simulink library "magnetometer_sim_lib"  (R2018b)
settings: Solver=VariableStepAuto  StartTime=0.0  StopTime=10.0  RelTol=1e-3
undefined symbols (not defined in the file): sim_params
libraries: simulink x3, dspmathops x2, aerolibutil x1
settings Model: Creator=colem  LastModifiedBy=colem

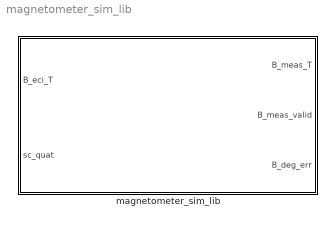
== system magnetometer_sim_lib ==
  magnetometer_sim_lib : Subsystem

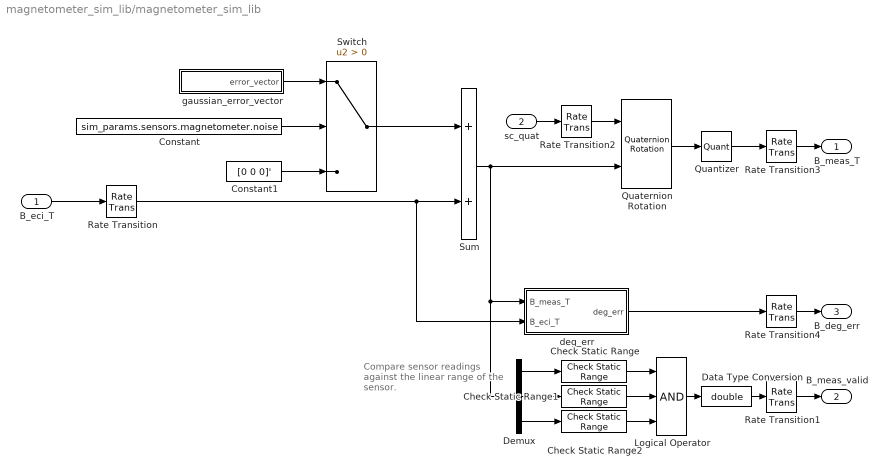
== system magnetometer_sim_lib/magnetometer_sim_lib ==
  note: Compare sensor readings
      | against the linear range
      | of the sensor.
  B_eci_T : Inport
  sc_quat : Inport  Port=2
  Check Static Range : simulink/Model Verification/Check  Static Range  Description=sim_params.sensors.magnetometer.B_min <= u <= sim_params.sensors.magnetometer.B_max  max=sim_params.sensors.magnetometer.B_max  max_included=on  min=sim_params.sensors.magnetometer.B_min  min_included=on  enabled=on  stopWhenAssertionFail=off  export=on  icon=text
      settings: SourceProductName=Simulink  SourceProductBaseCode=SL
  Check Static Range1 : simulink/Model Verification/Check  Static Range  Description=sim_params.sensors.magnetometer.B_min <= u <= sim_params.sensors.magnetometer.B_max  max=sim_params.sensors.magnetometer.B_max  max_included=on  min=sim_params.sensors.magnetometer.B_min  min_included=on  enabled=on  stopWhenAssertionFail=off  export=on  icon=graphic
      settings: SourceProductName=Simulink  SourceProductBaseCode=SL
  Check Static Range2 : simulink/Model Verification/Check  Static Range  Description=sim_params.sensors.magnetometer.B_min <= u <= sim_params.sensors.magnetometer.B_max  max=sim_params.sensors.magnetometer.B_max  max_included=on  min=sim_params.sensors.magnetometer.B_min  min_included=on  enabled=on  stopWhenAssertionFail=off  export=on  icon=graphic
      settings: SourceProductName=Simulink  SourceProductBaseCode=SL
  Constant : Constant  Value=sim_params.sensors.magnetometer.noise  SampleTime=sim_params.sensors.magnetometer.sample_time_s
  Constant1 : Constant  Value=[0 0 0]'  SampleTime=sim_params.sensors.magnetometer.sample_time_s
  Data Type Conversion : DataTypeConversion  OutDataTypeStr=double
  Demux : Demux  Outputs=3
  Logical Operator : Logic  Inputs=3  AllPortsSameDT=off  OutDataTypeStr=boolean
  Quantizer : Quantizer  QuantizationInterval=sim_params.sensors.magnetometer.resolution
  Quaternion Rotation : aerolibutil/Quaternion Rotation
  Rate Transition : RateTransition  InitialCondition=sim_params.environment.magnetic.ic.eci_T  OutPortSampleTime=sim_params.sensors.magnetometer.sample_time_s
  Rate Transition1 : RateTransition
  Rate Transition2 : RateTransition  InitialCondition=sim_params.dynamics.ic.quat_init  OutPortSampleTime=sim_params.sensors.magnetometer.sample_time_s
  Rate Transition3 : RateTransition  InitialCondition=sim_params.environment.magnetic.ic.eci_T
  Rate Transition4 : RateTransition
  Sum : Sum
  Switch : Switch  Criteria=u2 > Threshold
  deg_err : Subsystem
  gaussian_error_vector : Subsystem
  B_meas_T : Outport
  B_meas_valid : Outport  Port=2
  B_deg_err : Outport  Port=3
  wires:
  sc_quat/1 -> Rate Transition2/1
  Switch/1 -> Sum/1
  Constant/1 -> Switch/2
  Sum/1 -> Quaternion Rotation/2, deg_err/1(B_meas_T), Demux/1
  Constant1/1 -> Switch/3
  gaussian_error_vector/1(error_vector) -> Switch/1
  B_eci_T/1 -> Rate Transition/1
  deg_err/1(deg_err) -> Rate Transition4/1
  Rate Transition/1 -> deg_err/2(B_eci_T), Sum/2
  Rate Transition1/1 -> B_meas_valid/1
  Rate Transition2/1 -> Quaternion Rotation/1
  Rate Transition3/1 -> B_meas_T/1
  Quaternion Rotation/1 -> Quantizer/1
  Rate Transition4/1 -> B_deg_err/1
  Quantizer/1 -> Rate Transition3/1
  Demux/1 -> Check Static Range/1
  Demux/2 -> Check Static Range1/1
  Demux/3 -> Check Static Range2/1
  Check Static Range/1 -> Logical Operator/1
  Check Static Range1/1 -> Logical Operator/2
  Check Static Range2/1 -> Logical Operator/3
  Logical Operator/1 -> Data Type Conversion/1
  Data Type Conversion/1 -> Rate Transition1/1

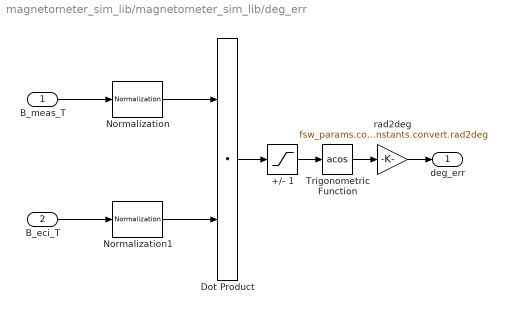
== system magnetometer_sim_lib/magnetometer_sim_lib/deg_err ==
  B_meas_T : Inport
  B_eci_T : Inport  Port=2
  +/- 1 : Saturate  UpperLimit=1  LowerLimit=-1
  Dot Product : DotProduct  InputSameDT=on  OutDataTypeStr=Inherit: Inherit via internal rule
  Normalization : dspmathops/Normalization  NormType=2-norm  Bias=1e-10  NormOver=Each column  Dimension=1  roundingMode=Floor  overflowMode=off  accumDataTypeStr=Inherit: Same as product output  accumLastDataTypeStr=Inherit: Same as product output  outputDataTypeStr=Inherit: Same as product output  outputMin=[]  outputMax=[]  outputLastDataTypeStr=Inherit: Same as product output
      settings: SourceProductName=DSP System Toolbox
  Normalization1 : dspmathops/Normalization  NormType=2-norm  Bias=1e-10  NormOver=Each column  Dimension=1  roundingMode=Floor  overflowMode=off  accumDataTypeStr=Inherit: Same as product output  accumLastDataTypeStr=Inherit: Same as product output  outputDataTypeStr=Inherit: Same as product output  outputMin=[]  outputMax=[]  outputLastDataTypeStr=Inherit: Same as product output
      settings: SourceProductName=DSP System Toolbox
  Trigonometric Function : Trigonometry  Operator=acos
  rad2deg : Gain  Gain=fsw_params.constants.convert.rad2deg
  deg_err : Outport
  wires:
  B_meas_T/1 -> Normalization/1
  Normalization/1 -> Dot Product/1
  B_eci_T/1 -> Normalization1/1
  Normalization1/1 -> Dot Product/2
  Dot Product/1 -> +/- 1/1
  Trigonometric Function/1 -> rad2deg/1
  +/- 1/1 -> Trigonometric Function/1
  rad2deg/1 -> deg_err/1

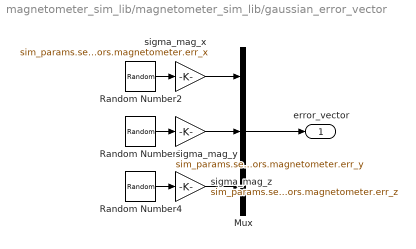
== system magnetometer_sim_lib/magnetometer_sim_lib/gaussian_error_vector ==
  Mux : Mux  Inputs=3
  Random Number2 : RandomNumber  Seed=4  SampleTime=sim_params.sensors.magnetometer.sample_time_s
  Random Number3 : RandomNumber  Seed=5  SampleTime=sim_params.sensors.magnetometer.sample_time_s
  Random Number4 : RandomNumber  Seed=6  SampleTime=sim_params.sensors.magnetometer.sample_time_s
  sigma_mag_x : Gain  Gain=sim_params.sensors.magnetometer.err_x
  sigma_mag_y : Gain  Gain=sim_params.sensors.magnetometer.err_y
  sigma_mag_z : Gain  Gain=sim_params.sensors.magnetometer.err_z
  error_vector : Outport
  wires:
  Random Number2/1 -> sigma_mag_x/1
  Random Number4/1 -> sigma_mag_z/1
  Random Number3/1 -> sigma_mag_y/1
  sigma_mag_x/1 -> Mux/1
  sigma_mag_y/1 -> Mux/2
  Mux/1 -> error_vector/1
  sigma_mag_z/1 -> Mux/3
